simulink model "abg_x_p2"  (R2014b)
settings: Solver=ode3  StartTime=0.0  StopTime=simtime  FixedStep=0.001  RelTol=1e-3
values from neighbouring files (symbols this model uses):
  a = 1    [path_config_cos.m]    (also in path_planning.m; path_planning_v0.m; path_planning_v1.m; path_planning_v2.m = 0.5)
  b = -1.5    [path_planning.m]    (also in path_planning_v1.m = 0; path_planning_v2.m = 0; run.m = -1; run_abg.m = 0)
  init_x_p = -9    [path_planning.m]    (also in path_planning_v0.m = -5; path_planning_v1.m = -6; path_planning_v2.m = 1; run.m = -5)
  init_x_p_dot = 0    [path_planning.m]    (also in path_planning_v0.m = 1; path_planning_v1.m = 10; path_planning_v2.m = 10; run.m)
  p = 0    [path_planning_v1.m]    (also in path_planning_v2.m = -2.5; run_abg.m; run_alpha.m = -2.5)
  w = pi/5    (= 0.628318530718)    [path_config_cos.m]    (also in path_planning.m; path_planning_v0.m; path_planning_v1.m; path_planning_v2.m = 0.314159265359)
settings Model: Creator=Fredrik  LastModifiedBy=Fredrik

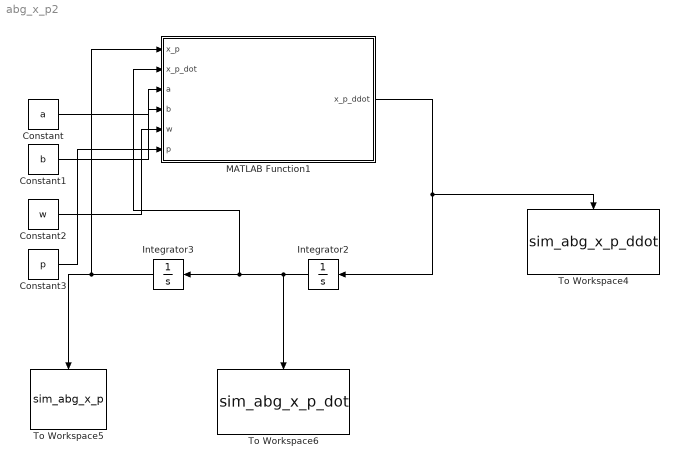
== system abg_x_p2 ==
  Constant : Constant  Value=a
  Constant1 : Constant  Value=b
  Constant2 : Constant  Value=w
  Constant3 : Constant  Value=p
  Integrator2 : Integrator  InitialCondition=init_x_p_dot
  Integrator3 : Integrator  InitialCondition=init_x_p
  MATLAB Function1 : MATLAB Function  TreatAsAtomicUnit=on
  To Workspace4 : ToWorkspace  VariableName=sim_abg_x_p_ddot  SaveFormat=Structure With Time  SampleTime=-1
  To Workspace5 : ToWorkspace  VariableName=sim_abg_x_p  SaveFormat=Structure With Time  SampleTime=-1
  To Workspace6 : ToWorkspace  VariableName=sim_abg_x_p_dot  SaveFormat=Structure With Time  SampleTime=-1
  wires:
  MATLAB Function1/1(x_p_ddot) -> To Workspace4/1, Integrator2/1
  Integrator3/1 -> MATLAB Function1/1(x_p), To Workspace5/1
  Integrator2/1 -> To Workspace6/1, MATLAB Function1/2(x_p_dot), Integrator3/1
  Constant/1 -> MATLAB Function1/3(a)
  Constant1/1 -> MATLAB Function1/4(b)
  Constant2/1 -> MATLAB Function1/5(w)
  Constant3/1 -> MATLAB Function1/6(p)

== matlab function abg_x_p2/MATLAB Function1 ==
  data: x_p input; x_p_ddot output; x_p_dot input; a input; b input; w input; p input
function x_p_ddot  = fcn(x_p, x_p_dot,a,b,w,p)
%#codegen

g=9.81;


%cos param v2

alfa = (1-(a*cos(w*x_p+p)+b)*a*sin(w*x_p+p)*w/sqrt(1-(a*cos(w*x_p+p)+b)^2))*(a*cos(w*x_p+p)+b)+(a*cos(w*x_p+p)+b)*a*sin(w*x_p+p)*w/(sqrt(1-(a*cos(w*x_p+p)+b)^2)*sqrt((a*cos(w*x_p+p)+b)^2));
beta = (((a*cos(w*x_p+p)+b)^2*a^2*sin(w*x_p+p)^2*w^2/(1-(a*cos(w*x_p+p)+b)^2)^(3/2)+a^2*sin(w*x_p+p)^2*w^2/sqrt(1-(a*cos(w*x_p+p)+b)^2)-(a*cos(w*x_p+p)+b)*a*cos(w*x_p+p)*w^2/sqrt(1-(a*cos(w*x_p+p)+b)^2))*(a*cos(w*x_p+p)+b)-(a*cos(w*x_p+p)+b)^2*a^2*sin(w*x_p+p)^2*w^2/((1-(a*cos(w*x_p+p)+b)^2)^(3/2)*sqrt((a*cos(w*x_p+p)+b)^2))-a^2*sin(w*x_p+p)^2*w^2/(sqrt(1-(a*cos(w*x_p+p)+b)^2)*sqrt((a*cos(w*x_p+p)+b)^2))+(a*cos(w*x_p+p)+b)*a*cos(w*x_p+p)*w^2/(sqrt(1-(a*cos(w*x_p+p)+b)^2)*sqrt((a*cos(w*x_p+p)+b)^2))+(a*cos(w*x_p+p)+b)^2*a^2*sin(w*x_p+p)^2*w^2/(sqrt(1-(a*cos(w*x_p+p)+b)^2)*((a*cos(w*x_p+p)+b)^2)^(3/2)));
gamma = -g*sqrt(1-(a*cos(w*x_p+p)+b)^2);


x_p_ddot = (-beta*(x_p_dot^2) - gamma)/alfa;
